simulink model "rtwdemo_advisor1"  (Simulink 6.0)
settings: Solver=VariableStepDiscrete  SolverMode=SingleTasking  StartTime=0.0  StopTime=4  FixedStep=1  RelTol=1e-3  AbsTol=1e-6
libraries: simulink x1, rtwdemowidgets x1
settings Model: CovMetricSettings=d  Creator=The MathWorks Inc.  LastModifiedBy=batserve  ExtModeTrigMode=oneshot  ExtModeArmWhenConnect=off  ExtModeAutoUpdateStatusClock=off  BufferReuse=off  ProdHWDeviceType=Specified
settings DataIOCC: LimitDataPoints=off  SaveFinalState=on  SaveOutput=off  SaveState=on  SignalLoggingName=sigsOut
settings OptimizationCC: BlockReduction=off  BooleanDataType=off  ConditionallyExecuteInputs=off  InlineInvariantSignals=off  OptimizeBlockIOStorage=off  BufferReuse=off  EnforceIntegerDowncast=off  ExpressionFolding=off  FoldNonRolledExpr=off  LocalBlockOutputs=off  ParameterPooling=off  OptimizeModelRefInitCode=on  LifeSpan=1
settings DebuggingCC: CheckExecutionContextPreStartOutputMsg=on  CheckExecutionContextRuntimeOutputMsg=on  SolverPrmCheckMsg=none  IntegerOverflowMsg=none  ParameterDowncastMsg=warning  ParameterOverflowMsg=warning  ParameterPrecisionLossMsg=none
settings HardwareCC: ProdBitPerInt=16  ProdHWDeviceType=Specified  TargetUnknown=on
settings RTWCC: SystemTargetFile=ert.tlc  GenCodeOnly=on  TemplateMakefile=ert_default_tmf  RTWVerbose=off  ProcessScript=ert_make_rtw_hook
settings CodeAppCC: GenerateComments=off  IgnoreCustomStorageClasses=off  IncHierarchyInIds=on  IncDataTypeInIds=on  SimulinkBlockComments=off
settings ERTTargetCC: TargetFcnLib=ansi_tfl_tmw.mat  GenFloatMathFcnCalls=ANSI_C  GenerateSampleERTMain=on  SupportContinuousTime=on  SupportNonInlinedSFcns=on  ExtMode=on  RootIOFormat=Individual Arguments  ERTCustomFileTemplate=example_file_process.tlc  InitialValueSource=Model

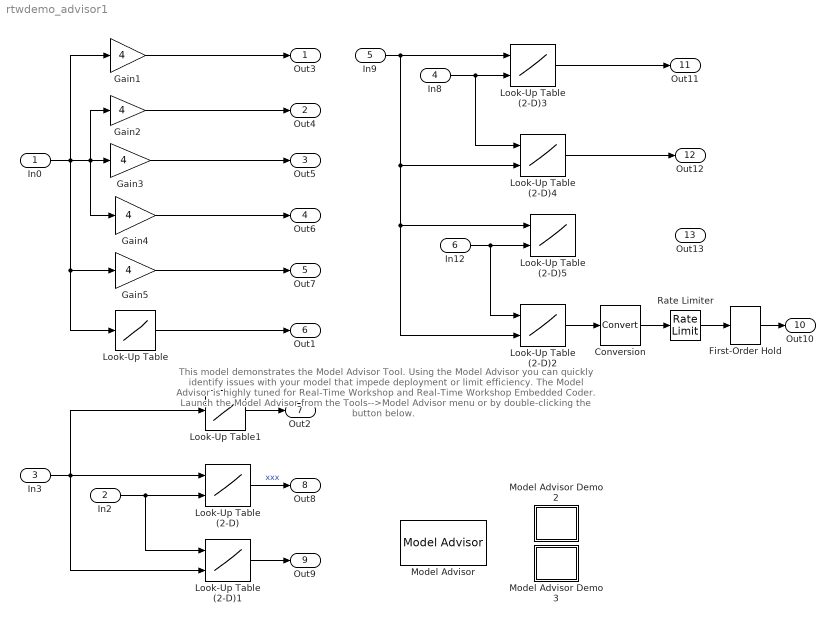
== system rtwdemo_advisor1 ==
  note: This model demonstrates the Model Advisor Tool.  Using the Model Advisor
      | you can quickly identify issues with your model that impede deployment
      | or limit efficiency.  The Model Advisor is highly tuned for Real-Time Workshop
      | and Real-Time Workshop Embedded Coder.  Launch the Model Advisor
      | from the Tools-->Model Advisor menu or by double-clicking the button below.
  In0 : Inport  Port=1  DataType=uint8  OutDataType=sfix(8)  OutScaling=2^-4  LatchInput=off  Interpolate=off
  In2 : Inport  Port=2  DataType=uint32  OutScaling=2^-10  LatchInput=off  Interpolate=off
  In3 : Inport  Port=3  DataType=uint32  OutScaling=2^-10  LatchInput=off  Interpolate=off
  In8 : Inport  Port=4  DataType=uint16  OutScaling=2^-10  LatchInput=off  Interpolate=off
  In9 : Inport  Port=5  DataType=uint16  OutScaling=2^-10  LatchInput=off  Interpolate=off
  In12 : Inport  Port=6  DataType=uint16  OutScaling=2^-10  LatchInput=off  Interpolate=off
  " Model Advisor Demo 2" : Subsystem  Orientation=up  PropExecContextAcrossSSBoundary=on
      settings: OpenFcn=rtwdemo_advisor2
      mask Display: disp('open')
  " Model Advisor Demo 3" : Subsystem  Orientation=up  PropExecContextAcrossSSBoundary=on
      settings: OpenFcn=rtwdemo_advisor3
      mask Display: disp('open')
  Conversion : DataTypeConversion  OutScaling=2^-10  ConvertRealWorld=Stored Integer (SI)
  First-Order Hold : simulink/Discrete/First-Order Hold  DisableCoverage=on  Ts=1
  Gain1 : Gain  Gain=4  ParameterScaling=2^-15  OutScaling=2^-10
  Gain2 : Gain  Gain=4  ParameterDataTypeMode=Specify via dialog  ParameterDataType=sfix(32)  ParameterScalingMode=Use specified scaling  OutScaling=2^-10  SaturateOnIntegerOverflow=on
  Gain3 : Gain  Gain=4  ParameterDataTypeMode=Specify via dialog  ParameterDataType=sfix(32)  ParameterScalingMode=Use specified scaling  OutScaling=2^-10
  Gain4 : Gain  Gain=4  ParameterDataTypeMode=Specify via dialog  ParameterDataType=sfix(32)  ParameterScalingMode=Use specified scaling  OutDataType=sfix(32)  OutScaling=2^-4
  Gain5 : Gain  Gain=4  ParameterDataTypeMode=Specify via dialog  ParameterDataType=sfix(32)  ParameterScalingMode=Use specified scaling  OutDataType=sfix(32)  OutScaling=2^-3  SaturateOnIntegerOverflow=on
  Look-Up Table : Lookup  DialogController=Simulink.DDGSource  InputValues=[0 1 3 7]  OutputValues=[9 3 9 3]  LookUpMeth=Interpolation-Use End Values  OutDataTypeMode=int16  OutScaling=2^-10  RndMeth=Nearest
  Look-Up Table (2-D) : Lookup2D  DialogController=Simulink.DDGSource  RowIndex=[1:3]  ColumnIndex=[1:3]  OutputValues=[4 5 6;16 19 20;10 18 23]  LookUpMeth=Interpolation-Use End Values  OutScaling=2^-10
  Look-Up Table (2-D)1 : Lookup2D  DialogController=Simulink.DDGSource  RowIndex=[0 2 5]  ColumnIndex=[1:3]  OutputValues=[4 5 6;16 19 20;10 18 23]  LookUpMeth=Interpolation-Use End Values  OutScaling=2^-10
  Look-Up Table (2-D)2 : Lookup2D  DialogController=Simulink.DDGSource  RowIndex=[1:3]  ColumnIndex=[1 2 7]  OutputValues=[4 5 6;16 19 20;10 18 23]  LookUpMeth=Interpolation-Use End Values  OutDataTypeMode=uint32  OutDataType=uint16(16)  OutScaling=2^-10
  Look-Up Table (2-D)3 : Lookup2D  DialogController=Simulink.DDGSource  RowIndex=[1:3]  ColumnIndex=[1:3]  OutputValues=[4 5 6;16 19 20;10 18 23]  LookUpMeth=Interpolation-Use End Values  OutScaling=2^-10
  Look-Up Table (2-D)4 : Lookup2D  DialogController=Simulink.DDGSource  RowIndex=[1:3]  ColumnIndex=[1 2 3 4 5]  OutputValues=ones(3,5)  LookUpMeth=Interpolation-Use End Values  OutDataTypeMode=uint16  OutScaling=2^-10
  Look-Up Table (2-D)5 : Lookup2D  DialogController=Simulink.DDGSource  RowIndex=[6 7 8 9 10]  ColumnIndex=[1:3]  OutputValues=ones(3,5).'  LookUpMeth=Interpolation-Use End Values  OutDataTypeMode=int16  OutScaling=2^-10
  Look-Up Table1 : Lookup  DialogController=Simulink.DDGSource  InputValues=[20 21 22 23 24]  OutputValues=[9 3 9 3 9]  LookUpMeth=Interpolation-Use End Values  OutDataTypeMode=uint16  OutScaling=2^-10
  Model Advisor : rtwdemowidgets/Model Advisor  attrib_overrides={}
  Rate Limiter : RateLimiter
  Out3 : Outport
  Out4 : Outport  Port=2
  Out5 : Outport  Port=3
  Out6 : Outport  Port=4
  Out7 : Outport  Port=5
  Out1 : Outport  Port=6
  Out2 : Outport  Port=7
  Out8 : Outport  Port=8
  Out9 : Outport  Port=9
  Out10 : Outport  Port=10
  Out11 : Outport  Port=11
  Out12 : Outport  Port=12
  Out13 : Outport  Port=13
  wires:
  Gain1/1 -> Out3/1
  Gain2/1 -> Out4/1
  Gain3/1 -> Out5/1
  Gain4/1 -> Out6/1
  Gain5/1 -> Out7/1
  Look-Up Table/1 -> Out1/1
  Look-Up Table1/1 -> Out2/1
  In2/1 -> Look-Up Table (2-D)/2, Look-Up Table (2-D)1/1
  Look-Up Table (2-D)/1 -> Out8/1  "xxx"
  In3/1 -> Look-Up Table (2-D)/1, Look-Up Table (2-D)1/2, Look-Up Table1/1
  Look-Up Table (2-D)1/1 -> Out9/1
  Look-Up Table (2-D)2/1 -> Conversion/1
  In8/1 -> Look-Up Table (2-D)4/1, Look-Up Table (2-D)3/2
  Look-Up Table (2-D)3/1 -> Out11/1
  In9/1 -> Look-Up Table (2-D)4/2, Look-Up Table (2-D)5/1, Look-Up Table (2-D)2/2, Look-Up Table (2-D)3/1
  Look-Up Table (2-D)4/1 -> Out12/1
  In12/1 -> Look-Up Table (2-D)5/2, Look-Up Table (2-D)2/1
  Rate Limiter/1 -> First-Order Hold/1
  Conversion/1 -> Rate Limiter/1
  First-Order Hold/1 -> Out10/1
  In0/1 -> Gain3/1, Gain4/1, Gain2/1, Gain1/1, Gain5/1, Look-Up Table/1

== system rtwdemo_advisor1/ Model Advisor Demo 2 ==

== system rtwdemo_advisor1/ Model Advisor Demo 3 ==
